simulink model "Avion_naturel_decouple"  (R2019b)
settings: Solver=VariableStepAuto  StartTime=0.0  StopTime=tsim  RelTol=1e-3
values from neighbouring files (symbols this model uses):
  A_simp = [-Xv -X_gamma 0 0 ... (first row only)    [Code_conduite_vol.m]
  B_simp = B_red    [Code_conduite_vol.m]
  C_simp = eye(4)    [Code_conduite_vol.m]
  D_simp = [0 0 0 0]'    [Code_conduite_vol.m]
  Kn_BdG = Wn_BdG^2*num_BdG    [Code_conduite_vol.m]
  Kq = 0.0785    [Code_conduite_vol.m]
  SW_BdG = 1    [Code_conduite_vol.m]
  SW_filtre = 1    [Code_conduite_vol.m]
  tau_filtre_q = mm/K    [Code_conduite_vol.m]
undefined symbols (not defined in the file or in its folder): den_BdG
settings Model: Creator=Alexa  LastModifiedBy=natha
settings DebuggingCC: SFMachineParentedDataDiag=error

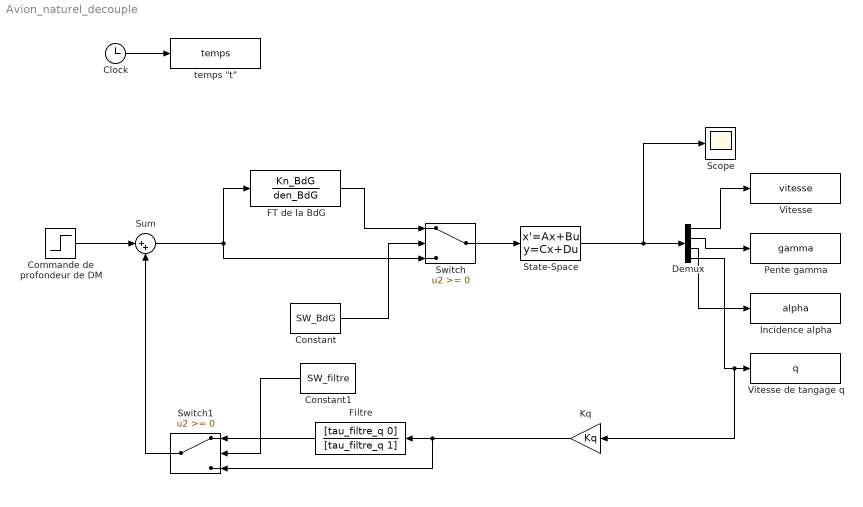
== system Avion_naturel_decouple ==
  Clock : Clock
  Commande de profondeur de DM : Step  Before=1  SampleTime=0
  Constant : Constant  Value=SW_BdG
  Constant1 : Constant  Value=SW_filtre
  Demux : Demux
  FT de la BdG : TransferFcn  Numerator=Kn_BdG  Denominator=den_BdG
  Filtre : TransferFcn  Numerator=[tau_filtre_q 0]  Denominator=[tau_filtre_q 1]
  Incidence alpha : ToWorkspace  VariableName=alpha  SampleTime=-1
  Kq : Gain  Gain=Kq
  Pente gamma : ToWorkspace  VariableName=gamma  SampleTime=-1
  Scope : Scope
  State-Space : StateSpace  A=A_simp  B=B_simp  C=C_simp  D=D_simp  InitialCondition=0
  Sum : Sum  Inputs=|++
  Switch : Switch
  Switch1 : Switch
  Vitesse : ToWorkspace  VariableName=vitesse  SampleTime=-1
  Vitesse de tangage q : ToWorkspace  VariableName=q  SampleTime=-1
  "temps \"t\"" : ToWorkspace  VariableName=temps  SampleTime=-1
  wires:
  Commande de profondeur de DM/1 -> Sum/1
  Switch/1 -> State-Space/1
  FT de la BdG/1 -> Switch/1
  Sum/1 -> FT de la BdG/1, Switch/3
  State-Space/1 -> Demux/1, Scope/1
  Constant/1 -> Switch/2
  Clock/1 -> "temps \"t\""/1
  Switch1/1 -> Sum/2
  Constant1/1 -> Switch1/2
  Filtre/1 -> Switch1/1
  Kq/1 -> Switch1/3, Filtre/1
  Demux/1 -> Vitesse/1
  Demux/2 -> Pente gamma/1
  Demux/3 -> Incidence alpha/1
  Demux/4 -> Kq/1, Vitesse de tangage q/1
